simulink model "satelita"  (R2016a)
settings: Solver=ode4  StartTime=0.0  StopTime=10.0  FixedStep=0.01  RelTol=1e-3
libraries: simulink x2
settings Model: Creator=ms36124  LastModifiedBy=ms36124

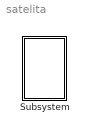
== system satelita ==
  Subsystem : Subsystem  mask{x=0, y=5, G=9.81, R=2, vx=10, M=100, rs=0.2, vy=0}

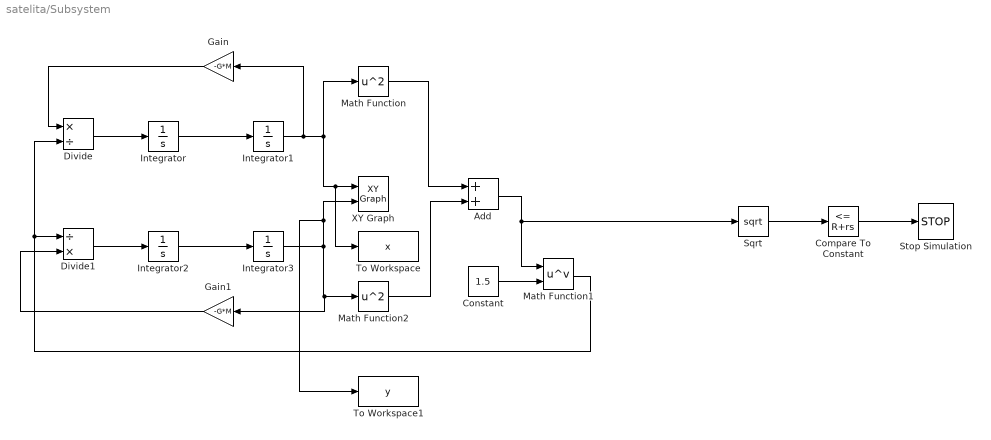
== system satelita/Subsystem ==
  Add : Sum
  Compare To Constant : simulink/Logic and Bit Operations/Compare To Constant  relop=<=  const=R+rs  OutDataTypeStr=boolean
  Constant : Constant  Value=1.5
  Divide : Product  Inputs=*/
  Divide1 : Product  Inputs=/*
  Gain : Gain  Gain=-G*M
  Gain1 : Gain  Gain=-G*M
  Integrator : Integrator  InitialCondition=vx
  Integrator1 : Integrator  InitialCondition=x
  Integrator2 : Integrator  InitialCondition=vy
  Integrator3 : Integrator  InitialCondition=y
  Math Function : Math  Operator=square  SaturateOnIntegerOverflow=on
  Math Function1 : Math  Operator=pow  SaturateOnIntegerOverflow=on
  Math Function2 : Math  Operator=square  SaturateOnIntegerOverflow=on
  Sqrt : Sqrt  SaturateOnIntegerOverflow=on
  Stop Simulation : Stop
  To Workspace : ToWorkspace  VariableName=x  SampleTime=-1
  To Workspace1 : ToWorkspace  VariableName=y  SampleTime=-1
  XY Graph : simulink/Sinks/XY Graph  xmin=-10  xmax=10  ymin=-10  ymax=10  st=-1
  wires:
  Integrator1/1 -> Gain/1, To Workspace/1, XY Graph/1, Math Function/1
  Divide/1 -> Integrator/1
  Add/1 -> Sqrt/1, Math Function1/1
  Integrator2/1 -> Integrator3/1
  Math Function1/1 -> Divide1/1, Divide/2
  Divide1/1 -> Integrator2/1
  Constant/1 -> Math Function1/2
  Integrator/1 -> Integrator1/1
  Gain/1 -> Divide/1
  Gain1/1 -> Divide1/2
  Math Function2/1 -> Add/2
  Math Function/1 -> Add/1
  Sqrt/1 -> Compare To Constant/1
  Compare To Constant/1 -> Stop Simulation/1
  Integrator3/1 -> Gain1/1, Math Function2/1, To Workspace1/1, XY Graph/2
